simulink model "Generation_de_trajectoire"  (R2018a)
settings: Solver=VariableStepAuto  StartTime=0.0  StopTime=10.0  RelTol=1e-3
values from neighbouring files (symbols this model uses):
  q_df = [ 0.00; 1.00;  0.00;  0.00;  0.00;  0.00]    [Q19Test.m]    (also in Q20Test.m)
  q_di = [-1.00; 0.00; -1.00; -1.00; -1.00; -1.00]    [Q19Test.m]    (also in Q20Test.m)
settings Model: Creator=Victor Kobayashi  LastModifiedBy=Victor Kobayashi

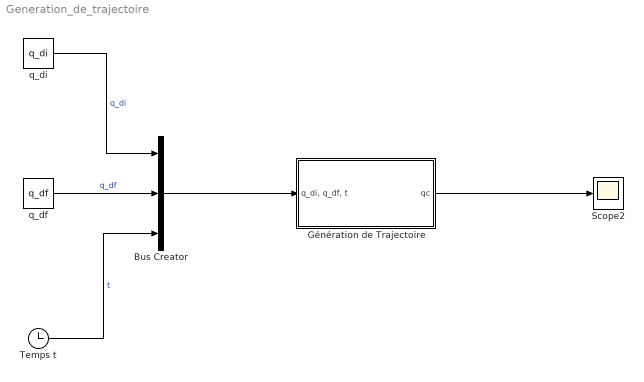
== system Generation_de_trajectoire ==
  Bus Creator : BusCreator  Inputs=3
  Génération de Trajectoire : Subsystem
  Scope2 : Scope
  "Temps t " : Clock
  "q_df " : Constant  Value=q_df
  q_di : Constant  Value=q_di
  wires:
  "q_df "/1 -> Bus Creator/2  "q_df"
  "Temps t "/1 -> Bus Creator/3  "t"
  q_di/1 -> Bus Creator/1  "q_di"
  Bus Creator/1 -> Génération de Trajectoire/1("q_di, q_df, t")
  Génération de Trajectoire/1(qc) -> Scope2/1

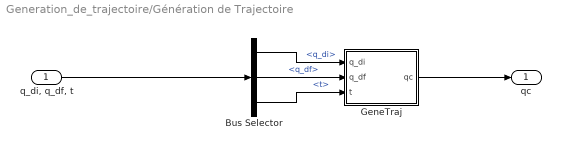
== system Generation_de_trajectoire/Génération de Trajectoire ==
  "q_di, q_df, t" : Inport
  Bus Selector : BusSelector  OutputSignals=q_di,q_df,t
  "GeneTraj " : MATLAB Function  TreatAsAtomicUnit=on
  qc : Outport
  wires:
  Bus Selector/3 -> "GeneTraj "/3(t)  "<t>"
  Bus Selector/1 -> "GeneTraj "/1(q_di)  "<q_di>"
  "q_di, q_df, t"/1 -> Bus Selector/1
  Bus Selector/2 -> "GeneTraj "/2(q_df)  "<q_df>"
  "GeneTraj "/1(qc) -> qc/1

== matlab function Generation_de_trajectoire/Génération de Trajectoire/GeneTraj  ==
  data: q_di input; qc output; q_df input; t input
function qc = fcn(q_di, q_df, t)

qc  = GeneTraj(q_di, q_df, t);
